simulink model "jacobian_transpose"  (R2019b)
settings: Solver=VariableStepAuto  StartTime=0.0  StopTime=4  RelTol=1e-3
undefined symbols (not defined in the file or in its folder): DiscIntNeverNeededParam, q0, Tc
settings Model: Creator=GA  LastModifiedBy=GA

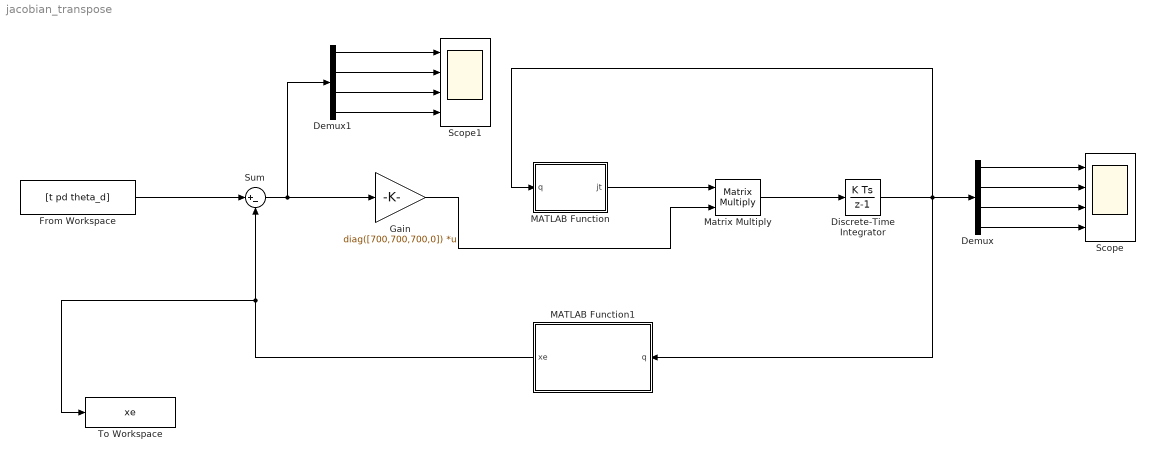
== system jacobian_transpose ==
  Demux : Demux
  Demux1 : Demux
  Discrete-Time Integrator : DiscreteIntegrator  gainval=1  InitialCondition=q0  SampleTime=Tc  ICPrevOutput=DiscIntNeverNeededParam  ICPrevScaledInput=DiscIntNeverNeededParam
  From Workspace : FromWorkspace  VariableName=[t pd theta_d]  SampleTime=0
  Gain : Gain  Gain=diag([700,700,700,0])  Multiplication=Matrix(K*u)
  MATLAB Function : MATLAB Function  TreatAsAtomicUnit=on
  MATLAB Function1 : MATLAB Function  TreatAsAtomicUnit=on
  Matrix Multiply : Product  Multiplication=Matrix(*)
  Scope : Scope  NumInputPorts=4
  Scope1 : Scope  NumInputPorts=4
  Sum : Sum  Inputs=|+-
  To Workspace : ToWorkspace  VariableName=xe  SaveFormat=Timeseries  SampleTime=-1
  wires:
  From Workspace/1 -> Sum/1
  Discrete-Time Integrator/1 -> MATLAB Function1/1(q), Demux/1, MATLAB Function/1(q)
  MATLAB Function/1(jt) -> Matrix Multiply/1
  Gain/1 -> Matrix Multiply/2
  Matrix Multiply/1 -> Discrete-Time Integrator/1
  Demux/4 -> Scope/4
  Demux/3 -> Scope/3
  Demux/1 -> Scope/1
  Demux/2 -> Scope/2
  Demux1/3 -> Scope1/3
  Demux1/1 -> Scope1/1
  Sum/1 -> Demux1/1, Gain/1
  Demux1/4 -> Scope1/4
  Demux1/2 -> Scope1/2
  MATLAB Function1/1(xe) -> To Workspace/1, Sum/2

== matlab function jacobian_transpose/MATLAB Function1 ==
  data: q input; xe output
function xe = non_linear_function(q)
a1 = 0.5;
a2 = 0.5;
d0 = 1;
xe = zeros(4,1);
xe(1,:) = a1*cos(q(1))+a2*cos(q(1)+q(2));
xe(2,:) = a1*sin(q(1))+a2*sin(q(1)+q(2));
xe(3,:) = d0 - q(3);
xe(4,:) = q(1)+q(2)+q(4);

== matlab function jacobian_transpose/MATLAB Function ==
  data: q input; jt output
function jt = fcn(q)

a1 = 0.5;
a2 = 0.5;

j = zeros(4,4);
j(1,1) = -a1*sin(q(1))-a2*sin(q(1)+q(2));
j(1,2) = -a2*sin(q(1)+q(2));
j(2,1) = a1*cos(q(1))+a2*cos(q(1)+q(2));
j(2,2) = a2*cos(q(1)+q(2));
j(3,3) = -1;
j(4,1) = 1;
j(4,2) = 1;
j(4,4) = 1;
jt = j';
